simulink model "bs_2o_1"  (R2022b)
settings: Solver=ode4  StartTime=0.0  StopTime=10.0  FixedStep=0.01  RelTol=1e-3
settings Model: Creator=张倬境  LastModifiedBy=张倬境

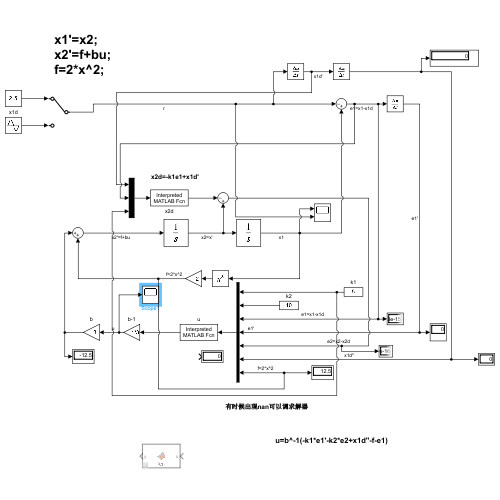
[thumbnail: Simulink's stored preview of the top-level diagram]
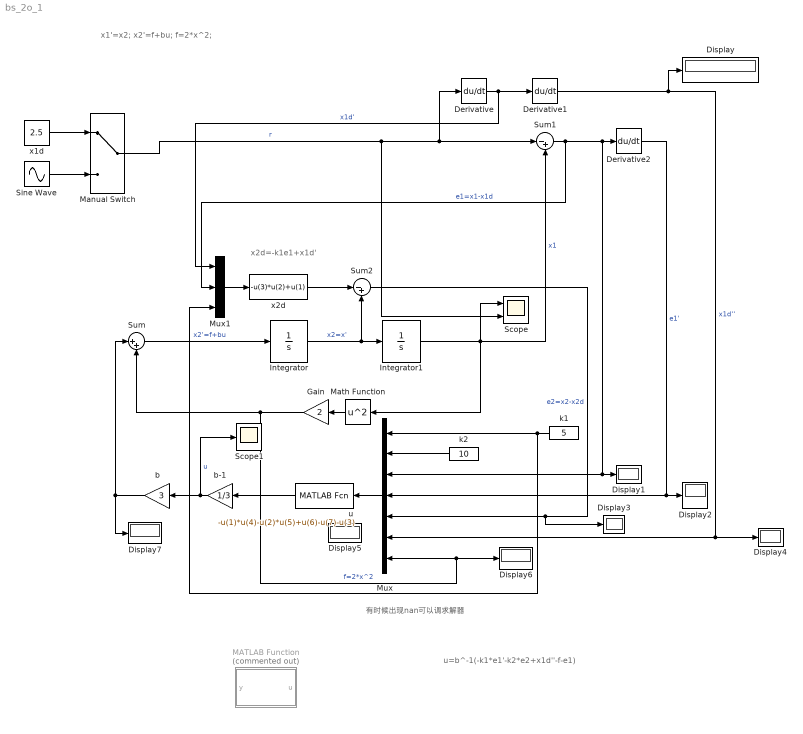
== system bs_2o_1 ==
  note: u=b^-1(-k1*e1'-k2*e2+x1d''-f-e1)
  note: 有时候出现nan可以调求解器
  note: x2d=-k1e1+x1d'
  note: x1'=x2;
      | x2'=f+bu;
      | f=2*x^2;
  Derivative : Derivative
  Derivative1 : Derivative
  Derivative2 : Derivative
  Display{,1..7} (8 alike) : Display
  Gain : Gain  Gain=2
  Integrator : Integrator
  Integrator1 : Integrator
  MATLAB Function : MATLAB Function  Commented=on  TreatAsAtomicUnit=on
  Manual Switch : ManualSwitch
  Math Function : Math  Operator=square
  Mux : Mux  Inputs=7
  Mux1 : Mux  Inputs=3
  Scope : Scope  NumInputPorts=2
  Scope1 : Scope
  Sine Wave : Sin  SampleTime=0
  Sum : Sum  Inputs=|++
  Sum1 : Sum  Inputs=|-+
  Sum2 : Sum  Inputs=|-+
  b : Gain  Gain=3
  b-1 : Gain  Gain=1/3
  k1 : Constant  Value=5
  k2 : Constant  Value=10
  u : MATLABFcn  MATLABFcn=-u(1)*u(4)-u(2)*u(5)+u(6)-u(7)-u(3)  OutputDimensions=[1 1]  OutputSignalType=real  Output1D=off
  x1d : Constant  Value=2.5
  x2d : MATLABFcn  MATLABFcn=-u(3)*u(2)+u(1)
  wires:
  Integrator1/1 -> Scope/1, Sum1/2, Math Function/1  "x1"
  Integrator/1 -> Sum2/2, Integrator1/1  "x2=x'"
  Math Function/1 -> Gain/1
  Sum/1 -> Integrator/1  "x2'=f+bu"
  Gain/1 -> Mux/7, Display6/1, Sum/2  "f=2*x^2"
  b/1 -> Display7/1, Sum/1
  Derivative/1 -> Mux1/1, Derivative1/1  "x1d'"
  Sum1/1 -> Mux1/2, Derivative2/1, Mux/3, Display1/1  "e1=x1-x1d"
  b-1/1 -> Scope1/1, b/1  "u"
  k2/1 -> Mux/2
  Derivative2/1 -> Mux/4, Display2/1  "e1'"
  Derivative1/1 -> Display/1, Display4/1, Mux/6  "x1d''"
  x2d/1 -> Sum2/1
  Mux1/1 -> x2d/1
  k1/1 -> Mux1/3, Mux/1
  Sum2/1 -> Display3/1, Mux/5  "e2=x2-x2d"
  Sine Wave/1 -> Manual Switch/2
  Manual Switch/1 -> Scope/2, Derivative/1, Sum1/1  "r"
  x1d/1 -> Manual Switch/1
  Mux/1 -> u/1
  u/1 -> b-1/1

== matlab function bs_2o_1/MATLAB Function ==
  data: u input; y output
function y = fcn(u)
y=-u(1)*u(4)-u(2)*u(5)+u(6)-u(7)-u(3);
